simulink model "ES004A_PwrUpSeq"  (R2013b)
settings: Solver=FixedStepDiscrete  SolverMode=SingleTasking  StartTime=0.0  StopTime=1  FixedStep=0.002  RelTol=1e-3
undefined symbols (not defined in the file): ELECGLBPRM_STRTUPSTCURRMEASWRMININTESTSTRT_CNT_U08, ELECGLBPRM_STRTUPSTDI_CNT_U08, ELECGLBPRM_STRTUPSTFLSMEMININSTRT_CNT_U08, ELECGLBPRM_STRTUPSTMTRDRVRININSTRT_CNT_U08, ELECGLBPRM_STRTUPSTPWRDISCNCTATESTSTRT_CNT_U08, ELECGLBPRM_STRTUPSTPWRDISCNCTBTESTSTRT_CNT_U08, ELECGLBPRM_STRTUPSTTMPLMONININTESTSTRT_CNT_U08, ELECGLBPRM_STRTUPSTWARMININCMPL_CNT_U08, PWRTURNOFFCTRLTHD_CNT_U08, sigbuilder_block
libraries: simulink x3
(part 1 of 2)
settings Model: Creator=BZ9NJH  LastModifiedBy=TZBSJD
settings SolverCC: AutoInsertRateTranBlk=on  InsertRTBMode=Always
settings DataIOCC: LimitDataPoints=off  SaveFormat=Structure  ReturnWorkspaceOutputs=on
settings OptimizationCC: BlockReduction=off  InlineParams=on  ZeroExternalMemoryAtStartup=off  ZeroInternalMemoryAtStartup=off  OptimizeModelRefInitCode=on  LifeSpan=1
settings DebuggingCC: SignalInfNanChecking=error  SignalRangeChecking=warning  UnderspecifiedInitializationDetection=Simplified  SolverPrmCheckMsg=error  InheritedTsInSrcMsg=error  DiscreteInheritContinuousMsg=error  SingleTaskRateTransMsg=error  TasksWithSamePriorityMsg=error  SigSpecEnsureSampleTimeMsg=error  CheckMatrixSingularityMsg=error  IntegerOverflowMsg=none  ParameterUnderflowMsg=error  ParameterPrecisionLossMsg=error  ParameterTunabilityLossMsg=error  FixptConstUnderflowMsg=warning  FixptConstOverflowMsg=warning  VectorMatrixConversionMsg=error  SignalLabelMismatchMsg=error  UnconnectedInputMsg=error  UnconnectedOutputMsg=error  UnconnectedLineMsg=error  SFcnCompatibilityMsg=error  UniqueDataStoreMsg=warning  BusObjectLabelMismatch=error  RootOutportRequireBusObject=error  AssertControl=DisableAll  ModelReferenceIOMsg=error  ModelReferenceVersionMismatchMessage=warning  ModelReferenceIOMismatchMessage=error  ModelReferenceCSMismatchMessage=warning  ModelReferenceDataLoggingMessage=error  StateNameClashWarn=warning  StrictBusMsg=ErrorOnBusTreatedAsVector  NonBusSignalsTreatedAsBus=error  SFUnexpectedBacktrackingDiag=error  SFInvalidInputDataAccessInChartInitDiag=error  SFNoUnconditionalDefaultTransitionDiag=error  SFTransitionOutsideNaturalParentDiag=error  SFUnconditionalTransitionShadowingDiag=error  SFUndirectedBroadcastEventsDiag=error
settings ModelReferenceCC: ModelReferenceNumInstancesAllowed=Single
settings RTWCC: SystemTargetFile=autosar.tlc  GenCodeOnly=on  TemplateMakefile=ert_default_tmf  Description=AUTOSAR  GenerateReport=on  ProcessScript=autosar_make_rtw_hook  LaunchReport=on
settings CodeAppCC: GenerateComments=off  IgnoreCustomStorageClasses=off  CustomSymbolStrType=$N$R$M  CustomSymbolStrBlkIO=$N$M  SimulinkBlockComments=off
settings STFCustomTargetCC: ParMdlRefBuildCompliant=on  CompOptLevelCompliant=on  IncludeMdlTerminateFcn=off  CombineOutputUpdateFcns=on  SuppressErrorStatus=on  ERTFirstTimeCompliant=on  ERTCustomFileBanners=on  SupportNonFinite=off  SupportComplex=off  SupportContinuousTime=off  SupportNonInlinedSFcns=off  MATLABClassNameForMDSCustomization=Simulink.SoftwareTarget.ERTCustomization  AutosarCompliant=on  GRTInterface=off  SystemTargetFile=autosar.tlc
settings ERTTargetCC: CodeReplacementLibrary=ANSI_C  ConcurrentExecutionCompliant=off  IncludeMdlTerminateFcn=off  SuppressErrorStatus=on  SupportNonFinite=off  SupportComplex=off  ModelStepFunctionPrototypeControlCompliant=off  CPPClassGenCompliant=off  AutosarCompliant=on  InlinedParameterPlacement=NonHierarchical  ERTCustomFileTemplate=example_file_process.tlc  EnableUserReplacementTypes=on

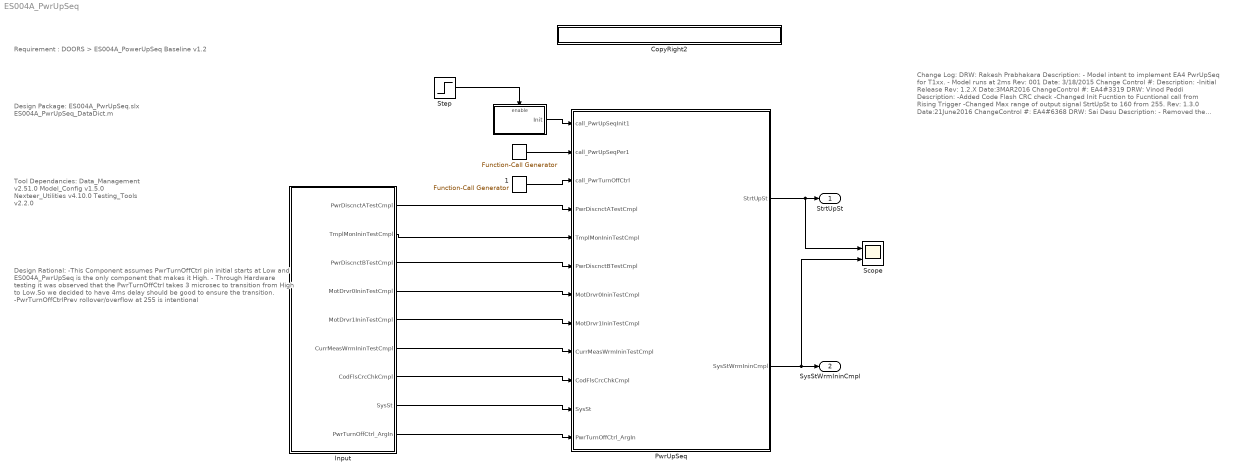
== system ES004A_PwrUpSeq ==
  note: Tool Dependancies:
      |
      | Data_Management v2.51.0
      | Model_Config v1.5.0
      | Nexteer_Utilities v4.10.0
      | Testing_Tools v2.2.0
  note: Design Package:
      |
      | ES004A_PwrUpSeq.slx
      | ES004A_PwrUpSeq_DataDict.m
  note: Requirement :
      |
      | DOORS > ES004A_PowerUpSeq Baseline v1.2
  note: Change Log:
      |
      | DRW: Rakesh Prabhakara
      | Description:
      | - Model intent to implement EA4 PwrUpSeq for T1xx.
      | - Model runs at 2ms
      |
      |
      | Rev: 001
      | Date: 3/18/2015
      | Change Control #:
      |
      | Description:
      | -Initial Release
      |
      | Rev: 1.2.X
      | Date:3MAR2016
      | ChangeControl #: EA4#3319
      | DRW: Vinod Peddi
      | Description:
      | -Added Code Flash CRC check
      | -Changed Init Fucntion to Fucntional call from Rising Trigger
      | -Changed Max range of output signal StrtUpSt to 160 from 255.
      |
      | Rev: 1.3.0
      | Date:21June2016
      | ChangeControl #: EA4#6368
      | DRW: Sai Desu
      | Description:
      | - Removed the StateFlow.
      |
      | Rev: 1.4.0
      | Date:7/12/2016
      | ChangeControl #: 	EA4#6487
      | DRW: Vinod Peddi
      | Description:
      | - Added MotDrv0IninTestCmpl and MotDrv1IninTestCmpl
      | -(Accounting for the changes in the Gate Drive FDDs)
      |
      | Rev: 1.5.0
      | Date:12/02/2016
      | ChangeControl #: 	EA4#8720
      | DRW: Sai Desu
      | Description:
      | - Added  logic in per1 to get TODpin to High state
      | - Added a new constant TURNOFFDLYTHD_CNT_U08 and new PIM PwrTurnOffCtrlPrev
      | -Added a new server for  PwrTurnOffCtrl pin control.
  note: Design Rational:
      | -This Component assumes PwrTurnOffCtrl pin
      | initial starts at Low and ES004A_PwrUpSeq
      | is the only component that makes it High.
      | - Through Hardware testing it was observed that
      | the PwrTurnOffCtrl takes 3 microsec to transition
      | from High to Low.So we decided to have 4ms delay
      | should be good to ensure the transition.
      | -PwrTurnOffCtrlPrev rollover/overflow at 255 is intentional
  "   " : simulink/Ports & Subsystems/Function-Call Generator  sample_time=0.002  numberOfIterations=1
  "    " : Subsystem  TreatAsAtomicUnit=on
  "   1" : simulink/Ports & Subsystems/Function-Call Generator  sample_time=0.002  numberOfIterations=1
  CopyRight2 : Subsystem  Description=|  mask(Copyright Information){none=on}
      | Copyright info block.                                               
      |                                                                     
      | Place copyright information at the top of every subsystem in design.
      mask prompts: none "No parameters"
      mask help: Place copyright information at the top of every subsystem in design.
      mask Display:
      | NxtrConf = 'Nexteer Confidential';
      | 
      | sys = bdroot; %handle for the current model ("system")
      | first = get_param(sys,'Created');
      | first = first(end-3:end);  %year is last four digits
      | 
      | last = get_param(sys,'LastModifiedDate');
      | if isempty(last)
      |     last = datestr(now,'yyyy');
      | else
      |     last = last(end-3:end);
      | end
      | 
      | if strcmp(first,last)
      |     fprintf('%s -- Copyright %s Nexteer',NxtrConf,first)
      | else
      |     fprintf('%s -- %s%s- %s Nexteer',NxtrConf,char(169),first,last)
      | end
  Input : Subsystem
      settings: AttributesFormatString=FOR SIMULATION ONLY
  PwrUpSeq : Subsystem  RequirementInfo={} %GIDa_35cfe924_8c92_4195_bef3_596e1ba51ef0
  Scope : Scope  NumInputPorts=2
      settings: YMin=-5~-5  YMax=5~5
  Step : Step  Before=1  After=0  SampleTime=0
  StrtUpSt : Outport
  SysStWrmIninCmpl : Outport  Port=2
  wires:
  "   "/1 -> PwrUpSeq/2(call_PwrUpSeqPer1)
  "    "/1(Init) -> PwrUpSeq/1(call_PwrUpSeqInit1)
  PwrUpSeq/1(StrtUpSt) -> StrtUpSt/1, Scope/1
  PwrUpSeq/2(SysStWrmIninCmpl) -> Scope/2, SysStWrmIninCmpl/1
  Step/1 -> "    "/Enable
  Input/1(PwrDiscnctATestCmpl) -> PwrUpSeq/4(PwrDiscnctATestCmpl)
  Input/2("TmplMonIninTestCmpl ") -> PwrUpSeq/5(TmplMonIninTestCmpl)
  Input/3(PwrDiscnctBTestCmpl) -> PwrUpSeq/6(PwrDiscnctBTestCmpl)
  Input/4(MotDrvr0IninTestCmpl) -> PwrUpSeq/7(MotDrvr0IninTestCmpl)
  Input/6(CurrMeasWrmIninTestCmpl) -> PwrUpSeq/9(CurrMeasWrmIninTestCmpl)
  Input/7(CodFlsCrcChkCmpl) -> PwrUpSeq/10(CodFlsCrcChkCmpl)
  Input/8(SysSt) -> PwrUpSeq/11(SysSt)
  Input/5(MotDrvr1IninTestCmpl) -> PwrUpSeq/8(MotDrvr1IninTestCmpl)
  "   1"/1 -> PwrUpSeq/3(call_PwrTurnOffCtrl)
  Input/9(PwrTurnOffCtrl_ArgIn) -> PwrUpSeq/12(PwrTurnOffCtrl_ArgIn)

== system ES004A_PwrUpSeq/     ==
  Enable : EnablePort
  CopyRight2 : Subsystem  Description=|  mask(Copyright Information){none=on}
      | Copyright info block.                                               
      |                                                                     
      | Place copyright information at the top of every subsystem in design.
      mask prompts: none "No parameters"
      mask help: Place copyright information at the top of every subsystem in design.
      mask Display:
      | NxtrConf = 'Nexteer Confidential';
      | 
      | sys = bdroot; %handle for the current model ("system")
      | first = get_param(sys,'Created');
      | first = first(end-3:end);  %year is last four digits
      | 
      | last = get_param(sys,'LastModifiedDate');
      | if isempty(last)
      |     last = datestr(now,'yyyy');
      | else
      |     last = last(end-3:end);
      | end
      | 
      | if strcmp(first,last)
      |     fprintf('%s -- Copyright %s Nexteer',NxtrConf,first)
      | else
      |     fprintf('%s -- %s%s- %s Nexteer',NxtrConf,char(169),first,last)
      | end
  call_GateDrvCtrlInit1 : simulink/Ports & Subsystems/Function-Call Generator  sample_time=0  numberOfIterations=1
  Init : Outport
  wires:
  call_GateDrvCtrlInit1/1 -> Init/1

== system ES004A_PwrUpSeq/CopyRight2 ==

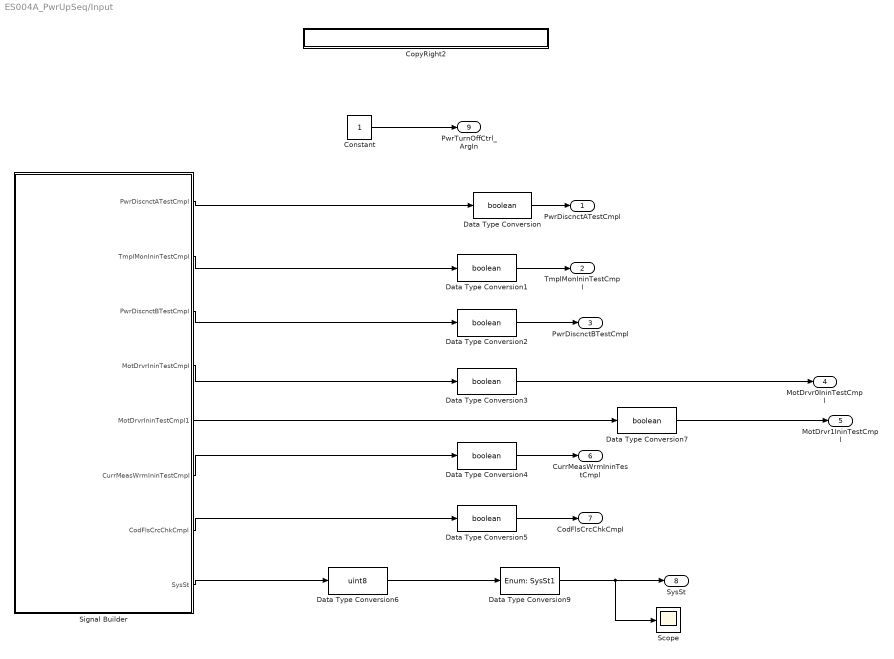
== system ES004A_PwrUpSeq/Input ==
  Constant : Constant  OutDataTypeStr=boolean
  CopyRight2 : Subsystem  Description=|  mask(Copyright Information){none=on}
      | Copyright info block.                                               
      |                                                                     
      | Place copyright information at the top of every subsystem in design.
      mask prompts: none "No parameters"
      mask help: Place copyright information at the top of every subsystem in design.
      mask Display:
      | NxtrConf = 'Nexteer Confidential';
      | 
      | sys = bdroot; %handle for the current model ("system")
      | first = get_param(sys,'Created');
      | first = first(end-3:end);  %year is last four digits
      | 
      | last = get_param(sys,'LastModifiedDate');
      | if isempty(last)
      |     last = datestr(now,'yyyy');
      | else
      |     last = last(end-3:end);
      | end
      | 
      | if strcmp(first,last)
      |     fprintf('%s -- Copyright %s Nexteer',NxtrConf,first)
      | else
      |     fprintf('%s -- %s%s- %s Nexteer',NxtrConf,char(169),first,last)
      | end
  Data Type Conversion{,1..5,7} (7 alike) : DataTypeConversion  OutDataTypeStr=boolean
  Data Type Conversion6 : DataTypeConversion  OutDataTypeStr=uint8
  Data Type Conversion9 : DataTypeConversion  OutDataTypeStr=Enum: SysSt1
      settings: AttributesFormatString=%<BlockType>
  Scope : Scope
  Signal Builder : Subsystem  Tag=STV Subsys  LoadFcn=sigbuilder_block('load');  StartFcn=sigbuilder_block('start');  StopFcn=sigbuilder_block('stop');  ClipboardFcn=sigbuilder_block('clipboard');  mask(Sigbuilder block){}
      mask help: Simulink:masks:SigbuilderBlock_MD
      mask init:
      | if ~strcmp(get_param(bdroot(gcbh),'SimulationStatus'),'stopped') tuvar = sigbuilder_block('maskInit'); end
      settings: CopyFcn=sigbuilder_block('copy');  DeleteFcn=sigbuilder_block('delete');  ModelCloseFcn=sigbuilder_block('modelClose');  PreSaveFcn=sigbuilder_block('preSave');  PauseFcn=sigbuilder_block('pause');  ContinueFcn=sigbuilder_block('continue');  NameChangeFcn=sigbuilder_block('namechange');  OpenFcn=sigbuilder_block('open',[-1024.5 11.25 1024.5 519 ]);  CloseFcn=sigbuilder_block('close');
      mask Display: plot(0, 0, 100, 100,[2, 2, 32, 32, 2], [68, 8, 8, 68, 68],[32, 2], [38, 38], [32, 19, 2],[53, 60, 44], [32, 17, 17, 2],[16, 16, 31, 31]);txt = getActiveGroup(gcbh);text(2, 100, txt,'verticalAlignment', 'top');
  PwrDiscnctATestCmpl : Outport
  "TmplMonIninTestCmpl " : Outport  Port=2
  PwrDiscnctBTestCmpl : Outport  Port=3
  MotDrvr0IninTestCmpl : Outport  Port=4
  MotDrvr1IninTestCmpl : Outport  Port=5
  CurrMeasWrmIninTestCmpl : Outport  Port=6
  CodFlsCrcChkCmpl : Outport  Port=7
  SysSt : Outport  Port=8
  PwrTurnOffCtrl_ArgIn : Outport  Port=9
  wires:
  Data Type Conversion/1 -> PwrDiscnctATestCmpl/1
  Data Type Conversion1/1 -> "TmplMonIninTestCmpl "/1
  Data Type Conversion2/1 -> PwrDiscnctBTestCmpl/1
  Data Type Conversion3/1 -> MotDrvr0IninTestCmpl/1
  Data Type Conversion4/1 -> CurrMeasWrmIninTestCmpl/1
  Data Type Conversion5/1 -> CodFlsCrcChkCmpl/1
  Data Type Conversion6/1 -> Data Type Conversion9/1
  Data Type Conversion9/1 -> Scope/1, SysSt/1
  Signal Builder/1(PwrDiscnctATestCmpl) -> Data Type Conversion/1
  Signal Builder/2(TmplMonIninTestCmpl) -> Data Type Conversion1/1
  Signal Builder/3(PwrDiscnctBTestCmpl) -> Data Type Conversion2/1
  Signal Builder/4(MotDrvrIninTestCmpl) -> Data Type Conversion3/1
  Signal Builder/6(CurrMeasWrmIninTestCmpl) -> Data Type Conversion4/1
  Signal Builder/7(CodFlsCrcChkCmpl) -> Data Type Conversion5/1
  Signal Builder/8(SysSt) -> Data Type Conversion6/1
  Signal Builder/5(MotDrvrIninTestCmpl1) -> Data Type Conversion7/1
  Data Type Conversion7/1 -> MotDrvr1IninTestCmpl/1
  Constant/1 -> PwrTurnOffCtrl_ArgIn/1

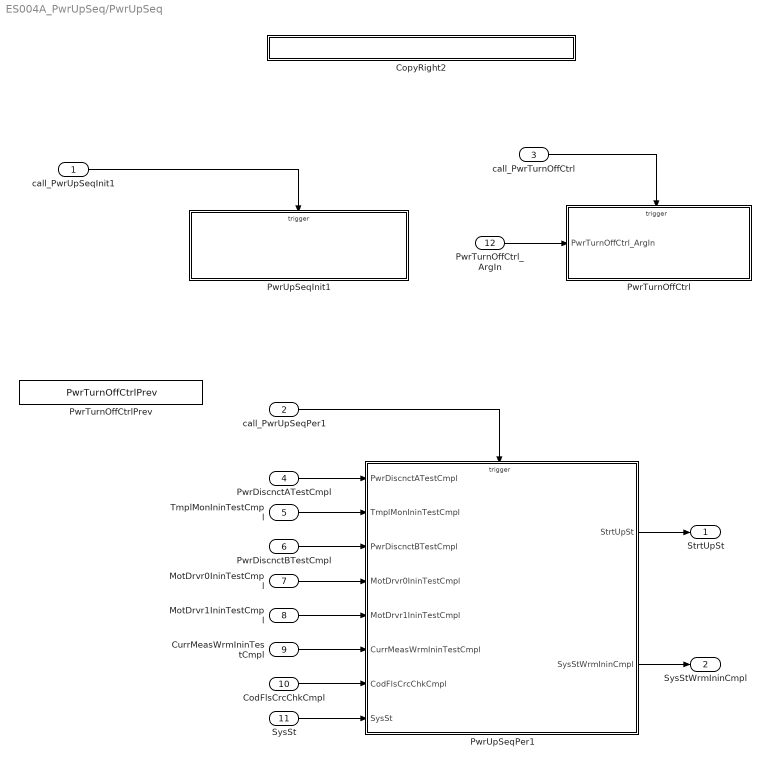
== system ES004A_PwrUpSeq/PwrUpSeq ==
  call_PwrUpSeqInit1 : Inport
  call_PwrUpSeqPer1 : Inport  Port=2
  call_PwrTurnOffCtrl : Inport  Port=3
  PwrDiscnctATestCmpl : Inport  RequirementInfo={} %GIDa_446bf28d_326e_4d71_9178_cb8879d17d30  Port=4
  TmplMonIninTestCmpl : Inport  RequirementInfo={} %GIDa_051ede06_809d_4a6b_ab11_6adf88300e4f  Port=5
  PwrDiscnctBTestCmpl : Inport  RequirementInfo={} %GIDa_4ad84e80_8ac9_4153_860d_30c67dab3eca  Port=6
  MotDrvr0IninTestCmpl : Inport  RequirementInfo={} %GIDa_14d41728_be18_48b9_a298_4b5d0108ece5  Port=7
  MotDrvr1IninTestCmpl : Inport  RequirementInfo="{}  %GIDa_c04dc9a0_694b_4c78_818e_03ab0f3abce0"  Port=8
  CurrMeasWrmIninTestCmpl : Inport  RequirementInfo={} %GIDa_d2f15d57_cae9_46da_aa94_3e87a93d3250  Port=9
  CodFlsCrcChkCmpl : Inport  RequirementInfo={} %GIDa_a8ee0d48_f2b0_430a_b961_b39c593c106a  Port=10
  SysSt : Inport  RequirementInfo={} %GIDa_cd61f2f6_0fac_48ad_93c3_ac49d9e424fd  Port=11
  PwrTurnOffCtrl_ArgIn : Inport  Port=12
  CopyRight2 : Subsystem  Description=|  mask(Copyright Information){none=on}
      | Copyright info block.                                               
      |                                                                     
      | Place copyright information at the top of every subsystem in design.
      mask prompts: none "No parameters"
      mask help: Place copyright information at the top of every subsystem in design.
      mask Display:
      | NxtrConf = 'Nexteer Confidential';
      | 
      | sys = bdroot; %handle for the current model ("system")
      | first = get_param(sys,'Created');
      | first = first(end-3:end);  %year is last four digits
      | 
      | last = get_param(sys,'LastModifiedDate');
      | if isempty(last)
      |     last = datestr(now,'yyyy');
      | else
      |     last = last(end-3:end);
      | end
      | 
      | if strcmp(first,last)
      |     fprintf('%s -- Copyright %s Nexteer',NxtrConf,first)
      | else
      |     fprintf('%s -- %s%s- %s Nexteer',NxtrConf,char(169),first,last)
      | end
  PwrTurnOffCtrl : Subsystem  RequirementInfo={} %GIDa_2ddf7215_35b5_4bad_85c7_079bbc552366
  PwrTurnOffCtrlPrev : DataStoreMemory  DataStoreName=PwrTurnOffCtrlPrev  StateMustResolveToSignalObject=on
  PwrUpSeqInit1 : Subsystem
  PwrUpSeqPer1 : Subsystem  TreatAsAtomicUnit=on
  StrtUpSt : Outport  RequirementInfo={} %GIDa_a09a46f2_e758_4418_b300_e7ddefb852d6
  SysStWrmIninCmpl : Outport  RequirementInfo={} %GIDa_a94a2f61_8623_40ca_87d4_e2cd322971b0  Port=2
  wires:
  call_PwrUpSeqPer1/1 -> PwrUpSeqPer1/Trigger
  TmplMonIninTestCmpl/1 -> PwrUpSeqPer1/2(TmplMonIninTestCmpl)
  PwrDiscnctATestCmpl/1 -> PwrUpSeqPer1/1(PwrDiscnctATestCmpl)
  PwrDiscnctBTestCmpl/1 -> PwrUpSeqPer1/3(PwrDiscnctBTestCmpl)
  MotDrvr0IninTestCmpl/1 -> PwrUpSeqPer1/4(MotDrvr0IninTestCmpl)
  PwrUpSeqPer1/2(SysStWrmIninCmpl) -> SysStWrmIninCmpl/1
  PwrUpSeqPer1/1(StrtUpSt) -> StrtUpSt/1
  CurrMeasWrmIninTestCmpl/1 -> PwrUpSeqPer1/6("CurrMeasWrmIninTestCmpl ")
  SysSt/1 -> PwrUpSeqPer1/8(SysSt)
  CodFlsCrcChkCmpl/1 -> PwrUpSeqPer1/7(CodFlsCrcChkCmpl)
  call_PwrUpSeqInit1/1 -> PwrUpSeqInit1/Trigger
  MotDrvr1IninTestCmpl/1 -> PwrUpSeqPer1/5(MotDrvr1IninTestCmpl)
  call_PwrTurnOffCtrl/1 -> PwrTurnOffCtrl/Trigger
  PwrTurnOffCtrl_ArgIn/1 -> PwrTurnOffCtrl/1(PwrTurnOffCtrl_ArgIn)

== system ES004A_PwrUpSeq/    /CopyRight2 ==

== system ES004A_PwrUpSeq/Input/CopyRight2 ==

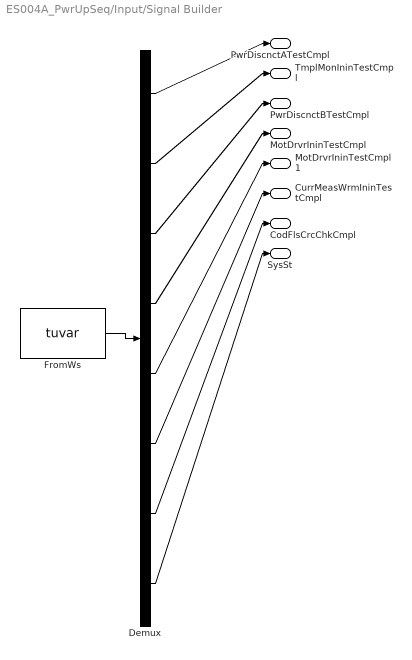
== system ES004A_PwrUpSeq/Input/Signal Builder ==
  Demux : Demux  Tag=STV Demux  Outputs=8
  FromWs : FromWorkspace  Tag=STV FromWs  VariableName=tuvar  SampleTime=0
      SigBuilderData=|
      | common.afterFinalStr = 'Extrapolate'
      | common.sampleTime = 0
      | dataSet(1).timeRange = [0 1]
      | dataSet(1).name = 'Ano Result'
      | dataSet(2).timeRange = [0 1]
      | dataSet(2).name = 'Loop Check'
      | dataSet(3).timeRange = [0 1]
      | dataSet(3).name = 'Loop Check1'
      | dataSet(4).timeRange = [0 1]
      | dataSet(4).name = 'Loop Check2'
      | sbobj.Groups(1).Name = 'Ano Result'
      | sbobj.Groups(1).Signals(1).Name = 'PwrDiscnctATestCmpl'
      | sbobj.Groups(1).Signals(1).XData = [0 0.19 0.62 1]
      | sbobj.Groups(1).Signals(1).YData = [1 1 1 1]
      | sbobj.Groups(1).Signals(2).Name = 'TmplMonIninTestCmpl'
      | sbobj.Groups(1).Signals(2).XData = [0 0.36 0.88 1]
      | sbobj.Groups(1).Signals(2).YData = [1 1 1 1]
      | sbobj.Groups(1).Signals(3).Name = 'PwrDiscnctBTestCmpl'
      | sbobj.Groups(1).Signals(3).XData = [0 0.53 1]
      | sbobj.Groups(1).Signals(3).YData = [1 1 1]
      | sbobj.Groups(1).Signals(4).Name = 'MotDrvrIninTestCmpl'
      | sbobj.Groups(1).Signals(4).XData = [0 0.7 1]
      | sbobj.Groups(1).Signals(4).YData = [1 1 1]
      | sbobj.Groups(1).Signals(5).Name = 'MotDrvrIninTestCmpl1'
      | sbobj.Groups(1).Signals(5).XData = [0 0.4 0.4 0.6 0.6 1]
      | sbobj.Groups(1).Signals(5).YData = [0 0 1 1 0 0]
      | sbobj.Groups(1).Signals(6).Name = 'CurrMeasWrmIninTestCmpl'
      | sbobj.Groups(1).Signals(6).XData = [0 0.92 1]
      | sbobj.Groups(1).Signals(6).YData = [1 1 1]
      | sbobj.Groups(1).Signals(7).Name = 'CodFlsCrcChkCmpl'
      | sbobj.Groups(1).Signals(7).XData = [0 1]
      | sbobj.Groups(1).Signals(7).YData = [1 1]
      | sbobj.Groups(1).Signals(8).Name = 'SysSt'
      | sbobj.Groups(1).Signals(8).XData = [0 1]
      | sbobj.Groups(1).Signals(8).YData = [3 3]
      | sbobj.Groups(1).TimeRange = [0 1]
      | sbobj.Groups(2).Name = 'Loop Check'
      | sbobj.Groups(2).Signals(1).Name = 'PwrDiscnctATestCmpl'
      | sbobj.Groups(2).Signals(1).XData = [0 0.078 0.078 0.156 0.156 0.19 0.62 1]
      | sbobj.Groups(2).Signals(1).YData = [1 1 0 0 1 1 1 1]
      | sbobj.Groups(2).Signals(2).Name = 'TmplMonIninTestCmpl'
      | sbobj.Groups(2).Signals(2).XData = [0 0.3 0.3 0.88 1]
      | sbobj.Groups(2).Signals(2).YData = [0 0 1 1 1]
      | sbobj.Groups(2).Signals(3).Name = 'PwrDiscnctBTestCmpl'
      | sbobj.Groups(2).Signals(3).XData = [0 0.4 0.4 1]
      | sbobj.Groups(2).Signals(3).YData = [0 0 1 1]
      | sbobj.Groups(2).Signals(4).Name = 'MotDrvrIninTestCmpl'
      | sbobj.Groups(2).Signals(4).XData = [0 0.501 0.501 1]
      | sbobj.Groups(2).Signals(4).YData = [0 0 1 1]
      | sbobj.Groups(2).Signals(5).Name = 'MotDrvrIninTestCmpl1'
      | sbobj.Groups(2).Signals(5).XData = [0 0.6 0.6 1]
      | sbobj.Groups(2).Signals(5).YData = [0 0 1 1]
      | sbobj.Groups(2).Signals(6).Name = 'CurrMeasWrmIninTestCmpl'
      | sbobj.Groups(2).Signals(6).XData = [0 0.7 0.7 1]
      | sbobj.Groups(2).Signals(6).YData = [0 0 1 1]
      | sbobj.Groups(2).Signals(7).Name = 'CodFlsCrcChkCmpl'
      | sbobj.Groups(2).Signals(7).XData = [0 0.8 0.8 1]
      | sbobj.Groups(2).Signals(7).YData = [0 0 1 1]
      | sbobj.Groups(2).Signals(8).Name = 'SysSt'
      | sbobj.Groups(2).Signals(8).XData = [0 0.045 0.045 0.098 0.098 0.331 0.331 0.359 0.359 0.522 0.522 0.562 0.562 1]
      | sbobj.Groups(2).Signals(8).YData = [0 0 1 1 3 3 1 1 3 3 2 2 3 3]
      | sbobj.Groups(2).TimeRange = [0 1]
      | sbobj.Groups(3).Name = 'Loop Check1'
      | sbobj.Groups(3).Signals(1).Name = 'PwrDiscnctATestCmpl'
      | sbobj.Groups(3).Signals(1).XData = [0 0.078 0.156 0.156 0.19 0.62 1]
      | sbobj.Groups(3).Signals(1).YData = [0 0 0 1 1 1 1]
      | sbobj.Groups(3).Signals(2).Name = 'TmplMonIninTestCmpl'
      | sbobj.Groups(3).Signals(2).XData = [0 0.2 0.2 0.88 1]
      | sbobj.Groups(3).Signals(2).YData = [0 0 1 1 1]
      | sbobj.Groups(3).Signals(3).Name = 'PwrDiscnctBTestCmpl'
      | sbobj.Groups(3).Signals(3).XData = [0 0.234 0.234 1]
      | sbobj.Groups(3).Signals(3).YData = [0 0 1 1]
      | sbobj.Groups(3).Signals(4).Name = 'MotDrvrIninTestCmpl'
      | sbobj.Groups(3).Signals(4).XData = [0 0.272 0.272 1]
      | sbobj.Groups(3).Signals(4).YData = [0 0 1 1]
      | sbobj.Groups(3).Signals(5).Name = 'MotDrvrIninTestCmpl1'
      | sbobj.Groups(3).Signals(5).XData = [0 0.274 1]
      | sbobj.Groups(3).Signals(5).YData = [0 0 0]
      | sbobj.Groups(3).Signals(6).Name = 'CurrMeasWrmIninTestCmpl'
      | sbobj.Groups(3).Signals(6).XData = [0 0.308 0.308 1]
      | sbobj.Groups(3).Signals(6).YData = [0 0 1 1]
      | sbobj.Groups(3).Signals(7).Name = 'CodFlsCrcChkCmpl'
      | sbobj.Groups(3).Signals(7).XData = [0 0.34 0.34 1]
      | sbobj.Groups(3).Signals(7).YData = [0 0 1 1]
      | sbobj.Groups(3).Signals(8).Name = 'SysSt'
      | sbobj.Groups(3).Signals(8).XData = [0 0.045 0.098 0.331 0.359 0.444 1]
      | sbobj.Groups(3).Signals(8).YData = [3 3 3 3 3 3 3]
      | sbobj.Groups(3).TimeRange = [0 1]
      | sbobj.Groups(4).Name = 'Loop Check2'
      | sbobj.Groups(4).Signals(1).Name = 'PwrDiscnctATestCmpl'
      | sbobj.Groups(4).Signals(1).XData = [0 0.078 0.156 0.156 0.19 0.62 1]
      | sbobj.Groups(4).Signals(1).YData = [0 0 0 1 1 1 1]
      | sbobj.Groups(4).Signals(2).Name = 'TmplMonIninTestCmpl'
      | sbobj.Groups(4).Signals(2).XData = [0 0.2 0.2 0.88 1]
      | sbobj.Groups(4).Signals(2).YData = [0 0 1 1 1]
      | sbobj.Groups(4).Signals(3).Name = 'PwrDiscnctBTestCmpl'
      | sbobj.Groups(4).Signals(3).XData = [0 0.234 0.234 1]
      | sbobj.Groups(4).Signals(3).YData = [0 0 1 1]
      | sbobj.Groups(4).Signals(4).Name = 'MotDrvrIninTestCmpl'
      | sbobj.Groups(4).Signals(4).XData = [0 0.272 0.272 1]
      | sbobj.Groups(4).Signals(4).YData = [0 0 1 1]
      | sbobj.Groups(4).Signals(5).Name = 'MotDrvrIninTestCmpl1'
      | sbobj.Groups(4).Signals(5).XData = [0 0.333 0.333 1]
      | sbobj.Groups(4).Signals(5).YData = [0 0 1 1]
      | sbobj.Groups(4).Signals(6).Name = 'CurrMeasWrmIninTestCmpl'
      | sbobj.Groups(4).Signals(6).XData = [0 0.308 0.308 1]
      | sbobj.Groups(4).Signals(6).YData = [0 0 1 1]
      | sbobj.Groups(4).Signals(7).Name = 'CodFlsCrcChkCmpl'
      | sbobj.Groups(4).Signals(7).XData = [0 0.34 0.34 1]
      | sbobj.Groups(4).Signals(7).YData = [0 0 1 1]
      | sbobj.Groups(4).Signals(8).Name = 'SysSt'
      | sbobj.Groups(4).Signals(8).XData = [0 0.045 0.098 0.331 0.359 0.359 0.444 0.444 1]
      | sbobj.Groups(4).Signals(8).YData = [3 3 3 3 3 0 0 2 2]
      | sbobj.Groups(4).TimeRange = [0 1]
  PwrDiscnctATestCmpl : Outport  Tag=STV Outport
  TmplMonIninTestCmpl : Outport  Tag=STV Outport  Port=2
  PwrDiscnctBTestCmpl : Outport  Tag=STV Outport  Port=3
  MotDrvrIninTestCmpl : Outport  Tag=STV Outport  Port=4
  MotDrvrIninTestCmpl1 : Outport  Tag=STV Outport  Port=5
  CurrMeasWrmIninTestCmpl : Outport  Tag=STV Outport  Port=6
  CodFlsCrcChkCmpl : Outport  Tag=STV Outport  Port=7
  SysSt : Outport  Tag=STV Outport  Port=8
  wires:
  FromWs/1 -> Demux/1
  Demux/1 -> PwrDiscnctATestCmpl/1
  Demux/2 -> TmplMonIninTestCmpl/1
  Demux/3 -> PwrDiscnctBTestCmpl/1
  Demux/4 -> MotDrvrIninTestCmpl/1
  Demux/5 -> MotDrvrIninTestCmpl1/1
  Demux/6 -> CurrMeasWrmIninTestCmpl/1
  Demux/7 -> CodFlsCrcChkCmpl/1
  Demux/8 -> SysSt/1

== system ES004A_PwrUpSeq/PwrUpSeq/CopyRight2 ==

== system ES004A_PwrUpSeq/PwrUpSeq/PwrTurnOffCtrl ==
  note: Note:
      | It is a function call for PIN P0_13
  PwrTurnOffCtrl_ArgIn : Inport
  function : TriggerPort  TriggerType=function-call
  CopyRight2 : Subsystem  Description=|  mask(Copyright Information){none=on}
      | Copyright info block.                                               
      |                                                                     
      | Place copyright information at the top of every subsystem in design.
      mask prompts: none "No parameters"
      mask help: Place copyright information at the top of every subsystem in design.
      mask Display:
      | NxtrConf = 'Nexteer Confidential';
      | 
      | sys = bdroot; %handle for the current model ("system")
      | first = get_param(sys,'Created');
      | first = first(end-3:end);  %year is last four digits
      | 
      | last = get_param(sys,'LastModifiedDate');
      | if isempty(last)
      |     last = datestr(now,'yyyy');
      | else
      |     last = last(end-3:end);
      | end
      | 
      | if strcmp(first,last)
      |     fprintf('%s -- Copyright %s Nexteer',NxtrConf,first)
      | else
      |     fprintf('%s -- %s%s- %s Nexteer',NxtrConf,char(169),first,last)
      | end
  IoHwAb_SetGpioPwrTurnOffCtrl : Subsystem  RequirementInfo={} %GIDa_63a85690_40db_495f_9f73_413351781123  TreatAsAtomicUnit=on
  wires:
  PwrTurnOffCtrl_ArgIn/1 -> IoHwAb_SetGpioPwrTurnOffCtrl/1(PinSt)

== system ES004A_PwrUpSeq/PwrUpSeq/PwrUpSeqInit1 ==
  note: Do Nothing
  function : TriggerPort  TriggerType=function-call
  CopyRight2 : Subsystem  Description=|  mask(Copyright Information){none=on}
      | Copyright info block.                                               
      |                                                                     
      | Place copyright information at the top of every subsystem in design.
      mask prompts: none "No parameters"
      mask help: Place copyright information at the top of every subsystem in design.
      mask Display:
      | NxtrConf = 'Nexteer Confidential';
      | 
      | sys = bdroot; %handle for the current model ("system")
      | first = get_param(sys,'Created');
      | first = first(end-3:end);  %year is last four digits
      | 
      | last = get_param(sys,'LastModifiedDate');
      | if isempty(last)
      |     last = datestr(now,'yyyy');
      | else
      |     last = last(end-3:end);
      | end
      | 
      | if strcmp(first,last)
      |     fprintf('%s -- Copyright %s Nexteer',NxtrConf,first)
      | else
      |     fprintf('%s -- %s%s- %s Nexteer',NxtrConf,char(169),first,last)
      | end

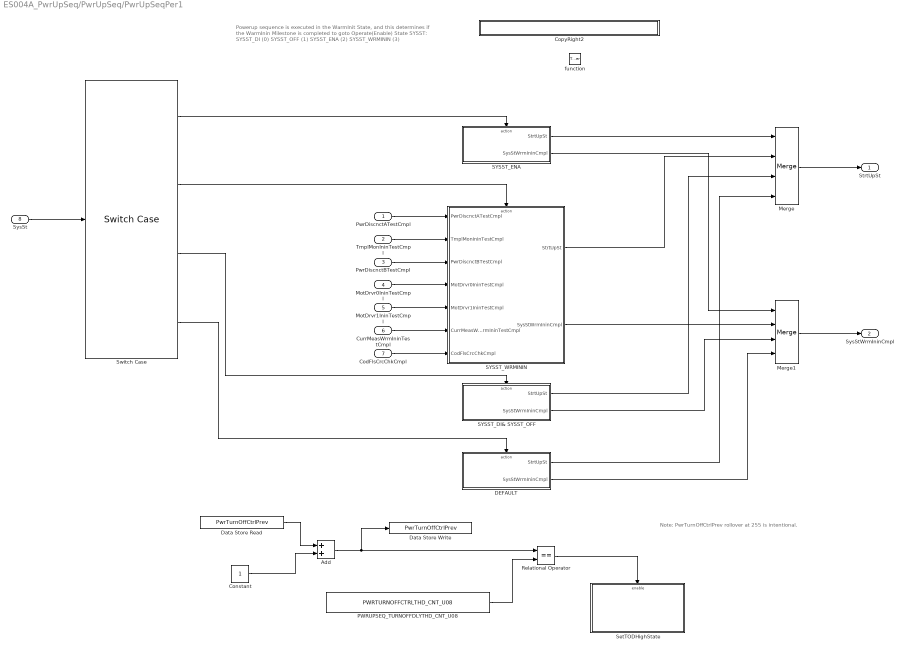
== system ES004A_PwrUpSeq/PwrUpSeq/PwrUpSeqPer1 ==
  note: Note:
      |       PwrTurnOffCtrlPrev rollover at 255 is intentional.
  note: Powerup sequence is executed in the WarmInit State, and this determines
      | if the WarmInin Milestone is completed to goto Operate(Enable) State
      |
      | SYSST:
      |         SYSST_DI               (0)
      |         SYSST_OFF            (1)
      |         SYSST_ENA            (2)
      |         SYSST_WRMININ   (3)
  PwrDiscnctATestCmpl : Inport
  TmplMonIninTestCmpl : Inport  Port=2
  PwrDiscnctBTestCmpl : Inport  Port=3
  MotDrvr0IninTestCmpl : Inport  Port=4
  MotDrvr1IninTestCmpl : Inport  Port=5
  "CurrMeasWrmIninTestCmpl " : Inport  Port=6
  CodFlsCrcChkCmpl : Inport  Port=7
  SysSt : Inport  Port=8
  function : TriggerPort  TriggerType=function-call
  Add : Sum
  Constant : Constant  OutDataTypeStr=uint8
  CopyRight2 : Subsystem  Description=|  mask(Copyright Information){none=on}
      | Copyright info block.                                               
      |                                                                     
      | Place copyright information at the top of every subsystem in design.
      mask prompts: none "No parameters"
      mask help: Place copyright information at the top of every subsystem in design.
      mask Display:
      | NxtrConf = 'Nexteer Confidential';
      | 
      | sys = bdroot; %handle for the current model ("system")
      | first = get_param(sys,'Created');
      | first = first(end-3:end);  %year is last four digits
      | 
      | last = get_param(sys,'LastModifiedDate');
      | if isempty(last)
      |     last = datestr(now,'yyyy');
      | else
      |     last = last(end-3:end);
      | end
      | 
      | if strcmp(first,last)
      |     fprintf('%s -- Copyright %s Nexteer',NxtrConf,first)
      | else
      |     fprintf('%s -- %s%s- %s Nexteer',NxtrConf,char(169),first,last)
      | end
  DEFAULT : Subsystem  TreatAsAtomicUnit=on
  Data Store Read : DataStoreRead  DataStoreName=PwrTurnOffCtrlPrev
  Data Store Write : DataStoreWrite  RequirementInfo={} %GIDa_df37f7ff_d87f_4e77_a2b4_f45c46094d7d  DataStoreName=PwrTurnOffCtrlPrev
  Merge : Merge  Inputs=4
  Merge1 : Merge  Inputs=4
  PWRUPSEQ_TURNOFFDLYTHD_CNT_U08 : Constant  Value=PWRTURNOFFCTRLTHD_CNT_U08
  Relational Operator : RelationalOperator  RequirementInfo={'linktype_rmi_doors' '0000c463 (/ESG Group/FDD Module Requirements/EA4 Specific/ES004A_PowerUpSeq)' '#ES004A_113' 'true' 'REQ: ES004A_113' '' } %GIDa_b6b0ea83_391c_4afc_bd1a_4830717992c4  Operator===  OutDataTypeStr=boolean
  SYSST_DI& SYSST_OFF : Subsystem  RequirementInfo="{'linktype_rmi_doors' '0000c463 (/ESG Group/FDD Module Requirements/EA4 Specific/ES004A_PowerUpSeq)' '#ES004A_84' 'true' 'REQ:  ES004A_84' '' } %GIDa_ceeac748_88a8_48cb_815e_66664c5915c7"  TreatAsAtomicUnit=on
  SYSST_ENA : Subsystem  TreatAsAtomicUnit=on
  SYSST_WRMININ : Subsystem  RequirementInfo="{'linktype_rmi_doors' '0000c463 (/ESG Group/FDD Module Requirements/EA4 Specific/ES004A_PowerUpSeq)' '#ES004A_82' 'true' 'REQ:  ES004A_82' '' } %GIDa_50562d96_a11b_4965_9ec2_ad4faf1a6e34"  TreatAsAtomicUnit=on
  "SetTODHighState " : Subsystem  RequirementInfo={'linktype_rmi_doors' '0000c463 (/ESG Group/FDD Module Requirements/EA4 Specific/ES004A_PowerUpSeq)' '#ES004A_113' 'true' 'REQ: ES004A_113' '' } %GIDa_db8fa826_8262_40dd_ba92_80414827086e
  Switch Case : SwitchCase  RequirementInfo="{'linktype_rmi_doors' '0000c463 (/ESG Group/FDD Module Requirements/EA4 Specific/ES004A_PowerUpSeq)' '#ES004A_84' 'true' 'REQ:  ES004A_84' '' } %GIDa_e0e763ba_a867_4216_bd03_69205a1b9b4f"  CaseConditions={SysSt1.SYSST_ENA,SysSt1.SYSST_WRMININ,[SysSt1.SYSST_DI,SysSt1.SYSST_OFF]}
  StrtUpSt : Outport
  SysStWrmIninCmpl : Outport  Port=2
  wires:
  SysSt/1 -> Switch Case/1
  Switch Case/1 -> SYSST_ENA/Action
  Switch Case/2 -> SYSST_WRMININ/Action
  PwrDiscnctATestCmpl/1 -> SYSST_WRMININ/1(PwrDiscnctATestCmpl)
  TmplMonIninTestCmpl/1 -> SYSST_WRMININ/2(TmplMonIninTestCmpl)
  PwrDiscnctBTestCmpl/1 -> SYSST_WRMININ/3(PwrDiscnctBTestCmpl)
  MotDrvr0IninTestCmpl/1 -> SYSST_WRMININ/4(MotDrvr0IninTestCmpl)
  "CurrMeasWrmIninTestCmpl "/1 -> SYSST_WRMININ/6("CurrMeasWrmIninTestCmpl ")
  CodFlsCrcChkCmpl/1 -> SYSST_WRMININ/7(CodFlsCrcChkCmpl)
  Switch Case/4 -> DEFAULT/Action
  Switch Case/3 -> SYSST_DI& SYSST_OFF/Action
  SYSST_WRMININ/1(StrtUpSt) -> Merge/2
  SYSST_ENA/1(StrtUpSt) -> Merge/1
  SYSST_ENA/2(SysStWrmIninCmpl) -> Merge1/1
  SYSST_WRMININ/2(SysStWrmIninCmpl) -> Merge1/2
  Merge/1 -> StrtUpSt/1
  Merge1/1 -> SysStWrmIninCmpl/1
  SYSST_DI& SYSST_OFF/1(StrtUpSt) -> Merge/3
  DEFAULT/1(StrtUpSt) -> Merge/4
  SYSST_DI& SYSST_OFF/2(SysStWrmIninCmpl) -> Merge1/3
  DEFAULT/2(SysStWrmIninCmpl) -> Merge1/4
  MotDrvr1IninTestCmpl/1 -> SYSST_WRMININ/5(MotDrvr1IninTestCmpl)
  Add/1 -> Relational Operator/1, Data Store Write/1
  Constant/1 -> Add/2
  Data Store Read/1 -> Add/1
  PWRUPSEQ_TURNOFFDLYTHD_CNT_U08/1 -> Relational Operator/2
  Relational Operator/1 -> "SetTODHighState "/Enable

== system ES004A_PwrUpSeq/PwrUpSeq/PwrTurnOffCtrl/CopyRight2 ==

== system ES004A_PwrUpSeq/PwrUpSeq/PwrTurnOffCtrl/IoHwAb_SetGpioPwrTurnOffCtrl ==
  PinSt : Inport  OutDataTypeStr=boolean
  CopyRight2 : Subsystem  Description=|  mask(Copyright Information){none=on}
      | Copyright info block.                                               
      |                                                                     
      | Place copyright information at the top of every subsystem in design.
      mask prompts: none "No parameters"
      mask help: Place copyright information at the top of every subsystem in design.
      mask Display:
      | NxtrConf = 'Nexteer Confidential';
      | 
      | sys = bdroot; %handle for the current model ("system")
      | first = get_param(sys,'Created');
      | first = first(end-3:end);  %year is last four digits
      | 
      | last = get_param(sys,'LastModifiedDate');
      | if isempty(last)
      |     last = datestr(now,'yyyy');
      | else
      |     last = last(end-3:end);
      | end
      | 
      | if strcmp(first,last)
      |     fprintf('%s -- Copyright %s Nexteer',NxtrConf,first)
      | else
      |     fprintf('%s -- %s%s- %s Nexteer',NxtrConf,char(169),first,last)
      | end
  Terminator : Terminator
  wires:
  PinSt/1 -> Terminator/1

== system ES004A_PwrUpSeq/PwrUpSeq/PwrUpSeqInit1/CopyRight2 ==

== system ES004A_PwrUpSeq/PwrUpSeq/PwrUpSeqPer1/CopyRight2 ==

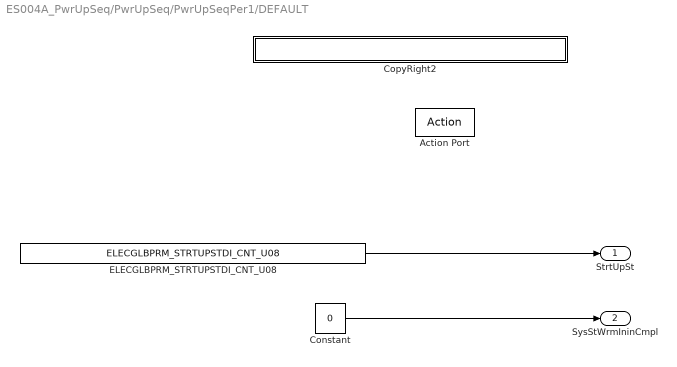
== system ES004A_PwrUpSeq/PwrUpSeq/PwrUpSeqPer1/DEFAULT ==
  Action Port : ActionPort  ActionType=default
  Constant : Constant  Value=0  OutDataTypeStr=boolean
  CopyRight2 : Subsystem  Description=|  mask(Copyright Information){none=on}
      | Copyright info block.                                               
      |                                                                     
      | Place copyright information at the top of every subsystem in design.
      mask prompts: none "No parameters"
      mask help: Place copyright information at the top of every subsystem in design.
      mask Display:
      | NxtrConf = 'Nexteer Confidential';
      | 
      | sys = bdroot; %handle for the current model ("system")
      | first = get_param(sys,'Created');
      | first = first(end-3:end);  %year is last four digits
      | 
      | last = get_param(sys,'LastModifiedDate');
      | if isempty(last)
      |     last = datestr(now,'yyyy');
      | else
      |     last = last(end-3:end);
      | end
      | 
      | if strcmp(first,last)
      |     fprintf('%s -- Copyright %s Nexteer',NxtrConf,first)
      | else
      |     fprintf('%s -- %s%s- %s Nexteer',NxtrConf,char(169),first,last)
      | end
  ELECGLBPRM_STRTUPSTDI_CNT_U08 : Constant  RequirementInfo="{'linktype_rmi_doors' '0000c463 (/ESG Group/FDD Module Requirements/EA4 Specific/ES004A_PowerUpSeq)' '#ES004A_92' 'true' 'REQ:  ES004A_92' '' } %GIDa_3597ee02_1051_49da_9cc1_a1bd3f94ea25"  Value=ELECGLBPRM_STRTUPSTDI_CNT_U08
  StrtUpSt : Outport
  SysStWrmIninCmpl : Outport  Port=2
  wires:
  Constant/1 -> SysStWrmIninCmpl/1
  ELECGLBPRM_STRTUPSTDI_CNT_U08/1 -> StrtUpSt/1

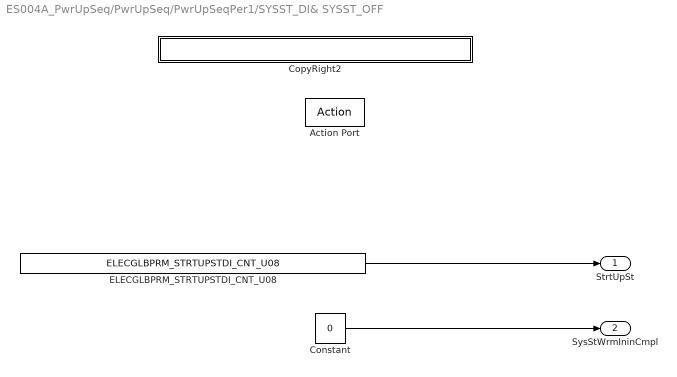
== system ES004A_PwrUpSeq/PwrUpSeq/PwrUpSeqPer1/SYSST_DI& SYSST_OFF ==
  Action Port : ActionPort  ActionType=case
  Constant : Constant  Value=0  OutDataTypeStr=boolean
  CopyRight2 : Subsystem  Description=|  mask(Copyright Information){none=on}
      | Copyright info block.                                               
      |                                                                     
      | Place copyright information at the top of every subsystem in design.
      mask prompts: none "No parameters"
      mask help: Place copyright information at the top of every subsystem in design.
      mask Display:
      | NxtrConf = 'Nexteer Confidential';
      | 
      | sys = bdroot; %handle for the current model ("system")
      | first = get_param(sys,'Created');
      | first = first(end-3:end);  %year is last four digits
      | 
      | last = get_param(sys,'LastModifiedDate');
      | if isempty(last)
      |     last = datestr(now,'yyyy');
      | else
      |     last = last(end-3:end);
      | end
      | 
      | if strcmp(first,last)
      |     fprintf('%s -- Copyright %s Nexteer',NxtrConf,first)
      | else
      |     fprintf('%s -- %s%s- %s Nexteer',NxtrConf,char(169),first,last)
      | end
  ELECGLBPRM_STRTUPSTDI_CNT_U08 : Constant  RequirementInfo="{'linktype_rmi_doors' '0000c463 (/ESG Group/FDD Module Requirements/EA4 Specific/ES004A_PowerUpSeq)' '#ES004A_92' 'true' 'REQ:  ES004A_92' '' } %GIDa_87f87ac4_a31d_47f8_aeca_77f2e092630c"  Value=ELECGLBPRM_STRTUPSTDI_CNT_U08
  StrtUpSt : Outport
  SysStWrmIninCmpl : Outport  Port=2
  wires:
  Constant/1 -> SysStWrmIninCmpl/1
  ELECGLBPRM_STRTUPSTDI_CNT_U08/1 -> StrtUpSt/1

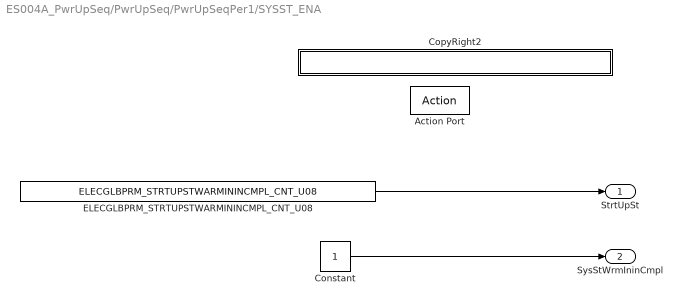
== system ES004A_PwrUpSeq/PwrUpSeq/PwrUpSeqPer1/SYSST_ENA ==
  Action Port : ActionPort  ActionType=case
  Constant : Constant  OutDataTypeStr=boolean
  CopyRight2 : Subsystem  Description=|  mask(Copyright Information){none=on}
      | Copyright info block.                                               
      |                                                                     
      | Place copyright information at the top of every subsystem in design.
      mask prompts: none "No parameters"
      mask help: Place copyright information at the top of every subsystem in design.
      mask Display:
      | NxtrConf = 'Nexteer Confidential';
      | 
      | sys = bdroot; %handle for the current model ("system")
      | first = get_param(sys,'Created');
      | first = first(end-3:end);  %year is last four digits
      | 
      | last = get_param(sys,'LastModifiedDate');
      | if isempty(last)
      |     last = datestr(now,'yyyy');
      | else
      |     last = last(end-3:end);
      | end
      | 
      | if strcmp(first,last)
      |     fprintf('%s -- Copyright %s Nexteer',NxtrConf,first)
      | else
      |     fprintf('%s -- %s%s- %s Nexteer',NxtrConf,char(169),first,last)
      | end
  ELECGLBPRM_STRTUPSTWARMININCMPL_CNT_U08 : Constant  RequirementInfo="{'linktype_rmi_doors' '0000c463 (/ESG Group/FDD Module Requirements/EA4 Specific/ES004A_PowerUpSeq)' '#ES004A_91' 'true' 'REQ:  ES004A_91' '' } %GIDa_1db9f596_d7fb_4f55_93ba_0bdf2c311370"  Value=ELECGLBPRM_STRTUPSTWARMININCMPL_CNT_U08
  StrtUpSt : Outport
  SysStWrmIninCmpl : Outport  Port=2
  wires:
  ELECGLBPRM_STRTUPSTWARMININCMPL_CNT_U08/1 -> StrtUpSt/1
  Constant/1 -> SysStWrmIninCmpl/1

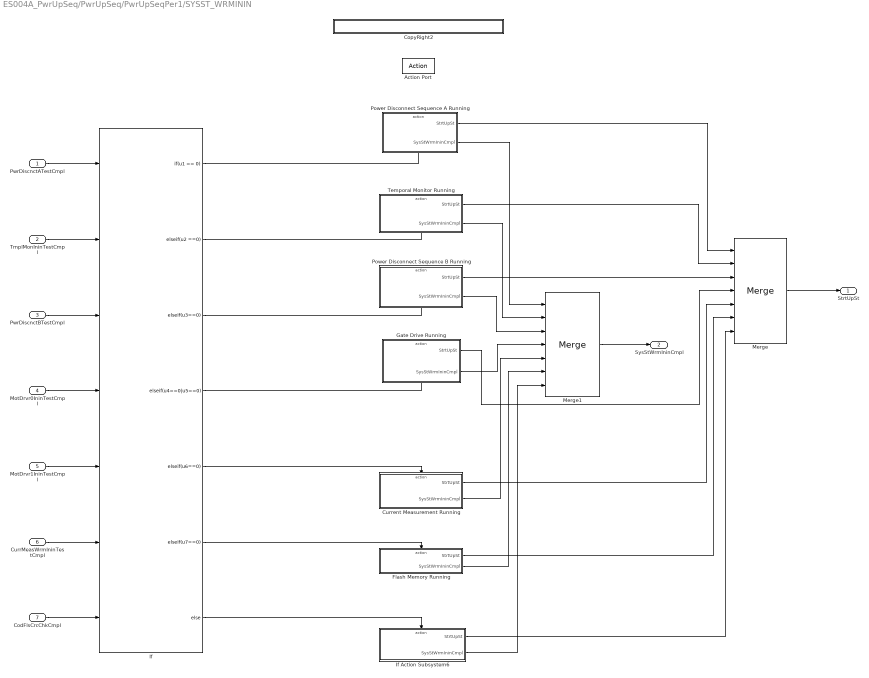
== system ES004A_PwrUpSeq/PwrUpSeq/PwrUpSeqPer1/SYSST_WRMININ ==
  PwrDiscnctATestCmpl : Inport
  TmplMonIninTestCmpl : Inport  Port=2
  PwrDiscnctBTestCmpl : Inport  Port=3
  MotDrvr0IninTestCmpl : Inport  Port=4
  MotDrvr1IninTestCmpl : Inport  Port=5
  "CurrMeasWrmIninTestCmpl " : Inport  Port=6
  CodFlsCrcChkCmpl : Inport  Port=7
  Action Port : ActionPort  ActionType=case
  CopyRight2 : Subsystem  Description=|  mask(Copyright Information){none=on}
      | Copyright info block.                                               
      |                                                                     
      | Place copyright information at the top of every subsystem in design.
      mask prompts: none "No parameters"
      mask help: Place copyright information at the top of every subsystem in design.
      mask Display:
      | NxtrConf = 'Nexteer Confidential';
      | 
      | sys = bdroot; %handle for the current model ("system")
      | first = get_param(sys,'Created');
      | first = first(end-3:end);  %year is last four digits
      | 
      | last = get_param(sys,'LastModifiedDate');
      | if isempty(last)
      |     last = datestr(now,'yyyy');
      | else
      |     last = last(end-3:end);
      | end
      | 
      | if strcmp(first,last)
      |     fprintf('%s -- Copyright %s Nexteer',NxtrConf,first)
      | else
      |     fprintf('%s -- %s%s- %s Nexteer',NxtrConf,char(169),first,last)
      | end
  Current Measurement Running : Subsystem  RequirementInfo="{'linktype_rmi_doors' '0000c463 (/ESG Group/FDD Module Requirements/EA4 Specific/ES004A_PowerUpSeq)' '#ES004A_81' 'true' 'REQ:  ES004A_81' '' } %GIDa_9127bcc1_cc29_496f_abb9_5387f3218dce"  TreatAsAtomicUnit=on
  Flash Memory Running : Subsystem  RequirementInfo="{'linktype_rmi_doors' '0000c463 (/ESG Group/FDD Module Requirements/EA4 Specific/ES004A_PowerUpSeq)' '#ES004A_83' 'true' 'REQ:  ES004A_83' '' } %GIDa_223a8b58_1f32_4b75_8519_612209f8a0b7"  TreatAsAtomicUnit=on
  Gate Drive Running : Subsystem  RequirementInfo="{'linktype_rmi_doors' '0000c463 (/ESG Group/FDD Module Requirements/EA4 Specific/ES004A_PowerUpSeq)' '#ES004A_79' 'true' 'REQ:  ES004A_79' '' } %GIDa_fa97780b_ce37_4938_a56c_a249d8282fc4"  TreatAsAtomicUnit=on
  If : If  RequirementInfo="{'linktype_rmi_doors' '0000c463 (/ESG Group/FDD Module Requirements/EA4 Specific/ES004A_PowerUpSeq)' '#ES004A_77' 'true' 'REQ:  ES004A_77' '' ; 'linktype_rmi_doors' '0000c463 (/ESG Group/FDD Module Requirements/EA4 Specific/ES004A_PowerUpSeq)' '#ES004A_78' 'true' 'REQ:  ES004A_78' '' ; 'linktype_rmi_doors' '0000c463 (/ESG Group/FDD Module Requirements/EA4 Specific/ES004A_PowerUpSeq)' '#ES004A_78' 'true' 'REQ:  ES004A_78' '' ; 'linktype_rmi_doors' '0000c463 (/ESG Group/FDD Module Requirements/EA4 Specific/ES004A_PowerUpSeq)' '#ES004A_79' 'true' 'REQ:  ES004A_79' '' ; 'linktype_rmi_doors' '0000c463 (/ESG Group/FDD Module Requirements/EA4 Specific/ES004A_PowerUpSeq)' '#ES004A_81' 'true' 'REQ:  ES004A_81' '' ; 'linktype_rmi_doors' '0000c463 (/ESG Group/FDD Module Requirements/EA4 Specific/ES004A_PowerUpSeq)' '#ES004A_83' 'true' 'REQ:  ES004A_83' '' ; 'linktype_rmi_doors' '0000c463 (/ESG Group/FDD Module Requirements/EA4 Specific/ES004A_PowerUpSeq)' '#ES004A_110' 'true' 'REQ:  ES004A_110' '' } %GIDa_cc1f6fd8_f4d8_407b_adba_65b9339b7100"  NumInputs=7  IfExpression=u1 == 0  ElseIfExpressions=u2 ==0 , u3==0 ,u4==0|u5==0,u6==0 ,u7==0
  If Action Subsystem6 : Subsystem  RequirementInfo="{'linktype_rmi_doors' '0000c463 (/ESG Group/FDD Module Requirements/EA4 Specific/ES004A_PowerUpSeq)' '#ES004A_110' 'true' 'REQ:  ES004A_110' '' } %GIDa_80ed37f1_ece5_4513_b447_e96ba05333ff"  TreatAsAtomicUnit=on
  Merge : Merge  RequirementInfo={} %GIDa_122839eb_5789_49ce_b5d2_bbf350e44528  Inputs=7
  Merge1 : Merge  RequirementInfo={} %GIDa_6a46f8bd_5f76_4d3c_9220_efb51c651a60  Inputs=7
  Power Disconnect Sequence A Running : Subsystem  RequirementInfo="{'linktype_rmi_doors' '0000c463 (/ESG Group/FDD Module Requirements/EA4 Specific/ES004A_PowerUpSeq)' '#ES004A_82' 'true' 'REQ:  ES004A_82' '' } %GIDa_c8935141_a908_4031_b016_5fc8ea4342bc"  TreatAsAtomicUnit=on
  Power Disconnect Sequence B Running : Subsystem  RequirementInfo="{'linktype_rmi_doors' '0000c463 (/ESG Group/FDD Module Requirements/EA4 Specific/ES004A_PowerUpSeq)' '#ES004A_78' 'true' 'REQ:  ES004A_78' '' } %GIDa_0ffc4163_1829_483d_be03_50a27c61aff4"  TreatAsAtomicUnit=on
  Temporal Monitor Running : Subsystem  RequirementInfo="{'linktype_rmi_doors' '0000c463 (/ESG Group/FDD Module Requirements/EA4 Specific/ES004A_PowerUpSeq)' '#ES004A_77' 'true' 'REQ:  ES004A_77' '' } %GIDa_acc93fdb_524a_4561_ac59_7d6169685fa0"  TreatAsAtomicUnit=on
  StrtUpSt : Outport  RequirementInfo="{'linktype_rmi_doors' '0000c463 (/ESG Group/FDD Module Requirements/EA4 Specific/ES004A_PowerUpSeq)' '#ES004A_55' 'true' 'REQ:  ES004A_55' '' } %GIDa_8fb86dbe_1acd_4e28_b2c1_efdddb0b395e"
  SysStWrmIninCmpl : Outport  Port=2
  wires:
  PwrDiscnctATestCmpl/1 -> If/1
  TmplMonIninTestCmpl/1 -> If/2
  PwrDiscnctBTestCmpl/1 -> If/3
  MotDrvr0IninTestCmpl/1 -> If/4
  "CurrMeasWrmIninTestCmpl "/1 -> If/6
  CodFlsCrcChkCmpl/1 -> If/7
  If/1 -> Power Disconnect Sequence A Running/Action
  If/2 -> Temporal Monitor Running/Action
  If/3 -> Power Disconnect Sequence B Running/Action
  If/4 -> Gate Drive Running/Action
  If/5 -> Current Measurement Running/Action
  If/6 -> Flash Memory Running/Action
  If/7 -> If Action Subsystem6/Action
  Merge1/1 -> SysStWrmIninCmpl/1
  Merge/1 -> StrtUpSt/1
  MotDrvr1IninTestCmpl/1 -> If/5
  Power Disconnect Sequence A Running/2(SysStWrmIninCmpl) -> Merge1/1
  Temporal Monitor Running/2(SysStWrmIninCmpl) -> Merge1/2
  Power Disconnect Sequence B Running/2(SysStWrmIninCmpl) -> Merge1/3
  Gate Drive Running/2(SysStWrmIninCmpl) -> Merge1/4
  Current Measurement Running/2(SysStWrmIninCmpl) -> Merge1/5
  Flash Memory Running/2(SysStWrmIninCmpl) -> Merge1/6
  If Action Subsystem6/2(SysStWrmIninCmpl) -> Merge1/7
  Power Disconnect Sequence A Running/1(StrtUpSt) -> Merge/1
  Temporal Monitor Running/1(StrtUpSt) -> Merge/2
  Power Disconnect Sequence B Running/1(StrtUpSt) -> Merge/3
  Gate Drive Running/1(StrtUpSt) -> Merge/4
  Current Measurement Running/1(StrtUpSt) -> Merge/5
  Flash Memory Running/1(StrtUpSt) -> Merge/6
  If Action Subsystem6/1(StrtUpSt) -> Merge/7

== system ES004A_PwrUpSeq/PwrUpSeq/PwrUpSeqPer1/SetTODHighState  ==
  note: Note:
      | PwrTurnOffCtrl is a SrvRunnable for thios component
      | so can be called as a local function in the software.
  Enable : EnablePort
  Constant : Constant  OutDataTypeStr=boolean
  CopyRight2 : Subsystem  Description=|  mask(Copyright Information){none=on}
      | Copyright info block.                                               
      |                                                                     
      | Place copyright information at the top of every subsystem in design.
      mask prompts: none "No parameters"
      mask help: Place copyright information at the top of every subsystem in design.
      mask Display:
      | NxtrConf = 'Nexteer Confidential';
      | 
      | sys = bdroot; %handle for the current model ("system")
      | first = get_param(sys,'Created');
      | first = first(end-3:end);  %year is last four digits
      | 
      | last = get_param(sys,'LastModifiedDate');
      | if isempty(last)
      |     last = datestr(now,'yyyy');
      | else
      |     last = last(end-3:end);
      | end
      | 
      | if strcmp(first,last)
      |     fprintf('%s -- Copyright %s Nexteer',NxtrConf,first)
      | else
      |     fprintf('%s -- %s%s- %s Nexteer',NxtrConf,char(169),first,last)
      | end
  PwrTurnOffCtrl : Subsystem  TreatAsAtomicUnit=on
  wires:
  Constant/1 -> PwrTurnOffCtrl/1(PwrTurnOffCtrl_ArgIn)

== system ES004A_PwrUpSeq/PwrUpSeq/PwrTurnOffCtrl/IoHwAb_SetGpioPwrTurnOffCtrl/CopyRight2 ==

== system ES004A_PwrUpSeq/PwrUpSeq/PwrUpSeqPer1/DEFAULT/CopyRight2 ==

== system ES004A_PwrUpSeq/PwrUpSeq/PwrUpSeqPer1/SYSST_DI& SYSST_OFF/CopyRight2 ==

== system ES004A_PwrUpSeq/PwrUpSeq/PwrUpSeqPer1/SYSST_ENA/CopyRight2 ==

== system ES004A_PwrUpSeq/PwrUpSeq/PwrUpSeqPer1/SYSST_WRMININ/CopyRight2 ==

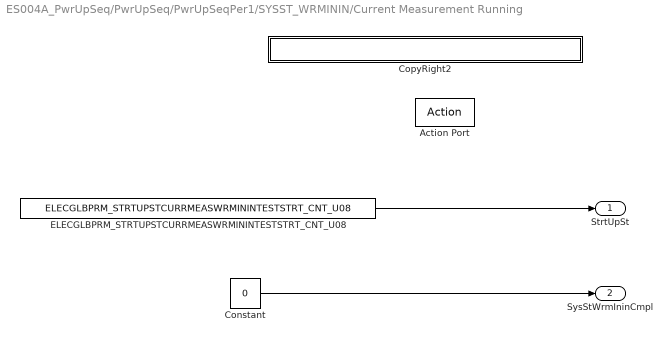
== system ES004A_PwrUpSeq/PwrUpSeq/PwrUpSeqPer1/SYSST_WRMININ/Current Measurement Running ==
  Action Port : ActionPort  ActionType=elseif
  Constant : Constant  Value=0  OutDataTypeStr=boolean
  CopyRight2 : Subsystem  Description=|  mask(Copyright Information){none=on}
      | Copyright info block.                                               
      |                                                                     
      | Place copyright information at the top of every subsystem in design.
      mask prompts: none "No parameters"
      mask help: Place copyright information at the top of every subsystem in design.
      mask Display:
      | NxtrConf = 'Nexteer Confidential';
      | 
      | sys = bdroot; %handle for the current model ("system")
      | first = get_param(sys,'Created');
      | first = first(end-3:end);  %year is last four digits
      | 
      | last = get_param(sys,'LastModifiedDate');
      | if isempty(last)
      |     last = datestr(now,'yyyy');
      | else
      |     last = last(end-3:end);
      | end
      | 
      | if strcmp(first,last)
      |     fprintf('%s -- Copyright %s Nexteer',NxtrConf,first)
      | else
      |     fprintf('%s -- %s%s- %s Nexteer',NxtrConf,char(169),first,last)
      | end
  ELECGLBPRM_STRTUPSTCURRMEASWRMININTESTSTRT_CNT_U08 : Constant  RequirementInfo="{'linktype_rmi_doors' '0000c463 (/ESG Group/FDD Module Requirements/EA4 Specific/ES004A_PowerUpSeq)' '#ES004A_90' 'true' 'REQ:  ES004A_90' '' } %GIDa_0e2887c5_0a04_45c7_936a_f5bd77c94aac"  Value=ELECGLBPRM_STRTUPSTCURRMEASWRMININTESTSTRT_CNT_U08
  StrtUpSt : Outport
  SysStWrmIninCmpl : Outport  Port=2
  wires:
  ELECGLBPRM_STRTUPSTCURRMEASWRMININTESTSTRT_CNT_U08/1 -> StrtUpSt/1
  Constant/1 -> SysStWrmIninCmpl/1

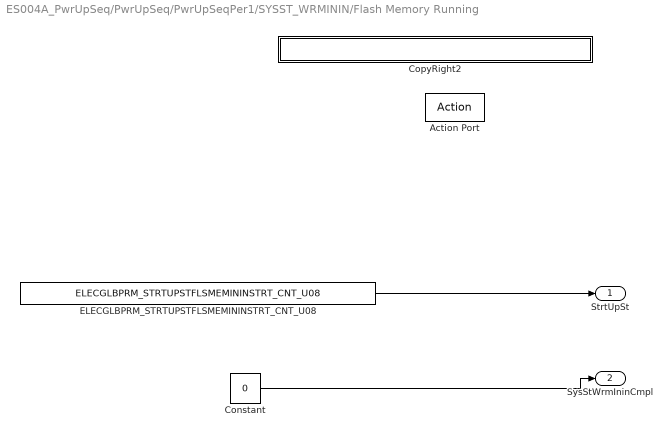
== system ES004A_PwrUpSeq/PwrUpSeq/PwrUpSeqPer1/SYSST_WRMININ/Flash Memory Running ==
  Action Port : ActionPort  ActionType=elseif
  Constant : Constant  Value=0  OutDataTypeStr=boolean
  CopyRight2 : Subsystem  Description=|  mask(Copyright Information){none=on}
      | Copyright info block.                                               
      |                                                                     
      | Place copyright information at the top of every subsystem in design.
      mask prompts: none "No parameters"
      mask help: Place copyright information at the top of every subsystem in design.
      mask Display:
      | NxtrConf = 'Nexteer Confidential';
      | 
      | sys = bdroot; %handle for the current model ("system")
      | first = get_param(sys,'Created');
      | first = first(end-3:end);  %year is last four digits
      | 
      | last = get_param(sys,'LastModifiedDate');
      | if isempty(last)
      |     last = datestr(now,'yyyy');
      | else
      |     last = last(end-3:end);
      | end
      | 
      | if strcmp(first,last)
      |     fprintf('%s -- Copyright %s Nexteer',NxtrConf,first)
      | else
      |     fprintf('%s -- %s%s- %s Nexteer',NxtrConf,char(169),first,last)
      | end
  ELECGLBPRM_STRTUPSTFLSMEMININSTRT_CNT_U08 : Constant  RequirementInfo="{'linktype_rmi_doors' '0000c463 (/ESG Group/FDD Module Requirements/EA4 Specific/ES004A_PowerUpSeq)' '#ES004A_105' 'true' 'REQ:  ES004A_105' '' } %GIDa_6d003dc2_d186_41c9_ae1c_92ef3d36c34c"  Value=ELECGLBPRM_STRTUPSTFLSMEMININSTRT_CNT_U08
  StrtUpSt : Outport
  SysStWrmIninCmpl : Outport  Port=2
  wires:
  ELECGLBPRM_STRTUPSTFLSMEMININSTRT_CNT_U08/1 -> StrtUpSt/1
  Constant/1 -> SysStWrmIninCmpl/1

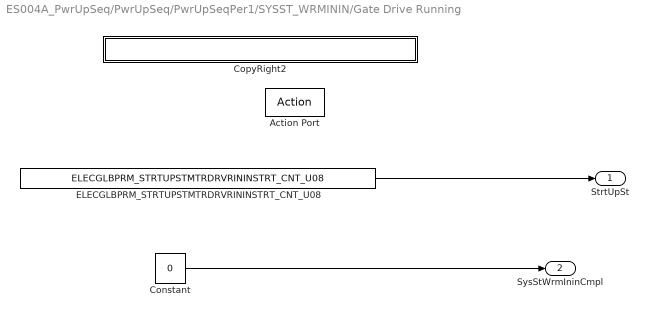
== system ES004A_PwrUpSeq/PwrUpSeq/PwrUpSeqPer1/SYSST_WRMININ/Gate Drive Running ==
  Action Port : ActionPort  ActionType=elseif
  Constant : Constant  Value=0  OutDataTypeStr=boolean
  CopyRight2 : Subsystem  Description=|  mask(Copyright Information){none=on}
      | Copyright info block.                                               
      |                                                                     
      | Place copyright information at the top of every subsystem in design.
      mask prompts: none "No parameters"
      mask help: Place copyright information at the top of every subsystem in design.
      mask Display:
      | NxtrConf = 'Nexteer Confidential';
      | 
      | sys = bdroot; %handle for the current model ("system")
      | first = get_param(sys,'Created');
      | first = first(end-3:end);  %year is last four digits
      | 
      | last = get_param(sys,'LastModifiedDate');
      | if isempty(last)
      |     last = datestr(now,'yyyy');
      | else
      |     last = last(end-3:end);
      | end
      | 
      | if strcmp(first,last)
      |     fprintf('%s -- Copyright %s Nexteer',NxtrConf,first)
      | else
      |     fprintf('%s -- %s%s- %s Nexteer',NxtrConf,char(169),first,last)
      | end
  ELECGLBPRM_STRTUPSTMTRDRVRININSTRT_CNT_U08 : Constant  RequirementInfo="{'linktype_rmi_doors' '0000c463 (/ESG Group/FDD Module Requirements/EA4 Specific/ES004A_PowerUpSeq)' '#ES004A_89' 'true' 'REQ:  ES004A_89' '' } %GIDa_36727618_0b71_4f5b_9cad_ec55d2d38298"  Value=ELECGLBPRM_STRTUPSTMTRDRVRININSTRT_CNT_U08
  StrtUpSt : Outport
  SysStWrmIninCmpl : Outport  Port=2
  wires:
  ELECGLBPRM_STRTUPSTMTRDRVRININSTRT_CNT_U08/1 -> StrtUpSt/1
  Constant/1 -> SysStWrmIninCmpl/1

== system ES004A_PwrUpSeq/PwrUpSeq/PwrUpSeqPer1/SYSST_WRMININ/If Action Subsystem6 ==
  Action Port : ActionPort  ActionType=else
  Constant : Constant  RequirementInfo="{'linktype_rmi_doors' '0000c463 (/ESG Group/FDD Module Requirements/EA4 Specific/ES004A_PowerUpSeq)' '#ES004A_62' 'true' 'REQ:  ES004A_62' '' } %GIDa_ef0c3e1b_e774_45f1_88e7_90c323b093a0"  OutDataTypeStr=boolean
  CopyRight2 : Subsystem  Description=|  mask(Copyright Information){none=on}
      | Copyright info block.                                               
      |                                                                     
      | Place copyright information at the top of every subsystem in design.
      mask prompts: none "No parameters"
      mask help: Place copyright information at the top of every subsystem in design.
      mask Display:
      | NxtrConf = 'Nexteer Confidential';
      | 
      | sys = bdroot; %handle for the current model ("system")
      | first = get_param(sys,'Created');
      | first = first(end-3:end);  %year is last four digits
      | 
      | last = get_param(sys,'LastModifiedDate');
      | if isempty(last)
      |     last = datestr(now,'yyyy');
      | else
      |     last = last(end-3:end);
      | end
      | 
      | if strcmp(first,last)
      |     fprintf('%s -- Copyright %s Nexteer',NxtrConf,first)
      | else
      |     fprintf('%s -- %s%s- %s Nexteer',NxtrConf,char(169),first,last)
      | end
  ELECGLBPRM_STRTUPSTWARMININCMPL_CNT_U08 : Constant  RequirementInfo="{'linktype_rmi_doors' '0000c463 (/ESG Group/FDD Module Requirements/EA4 Specific/ES004A_PowerUpSeq)' '#ES004A_91' 'true' 'REQ:  ES004A_91' '' } %GIDa_e5d51196_a843_4f31_946c_3457520e7be2"  Value=ELECGLBPRM_STRTUPSTWARMININCMPL_CNT_U08
  StrtUpSt : Outport
  SysStWrmIninCmpl : Outport  Port=2
  wires:
  ELECGLBPRM_STRTUPSTWARMININCMPL_CNT_U08/1 -> StrtUpSt/1
  Constant/1 -> SysStWrmIninCmpl/1

== system ES004A_PwrUpSeq/PwrUpSeq/PwrUpSeqPer1/SYSST_WRMININ/Power Disconnect Sequence A Running ==
  Action Port : ActionPort  ActionType=then
  Constant : Constant  RequirementInfo="{'linktype_rmi_doors' '0000c463 (/ESG Group/FDD Module Requirements/EA4 Specific/ES004A_PowerUpSeq)' '#ES004A_63' 'true' 'REQ:  ES004A_63' '' } %GIDa_1ac0845e_d558_4790_a0f1_f566be7b5692"  Value=0  OutDataTypeStr=boolean
  CopyRight2 : Subsystem  Description=|  mask(Copyright Information){none=on}
      | Copyright info block.                                               
      |                                                                     
      | Place copyright information at the top of every subsystem in design.
      mask prompts: none "No parameters"
      mask help: Place copyright information at the top of every subsystem in design.
      mask Display:
      | NxtrConf = 'Nexteer Confidential';
      | 
      | sys = bdroot; %handle for the current model ("system")
      | first = get_param(sys,'Created');
      | first = first(end-3:end);  %year is last four digits
      | 
      | last = get_param(sys,'LastModifiedDate');
      | if isempty(last)
      |     last = datestr(now,'yyyy');
      | else
      |     last = last(end-3:end);
      | end
      | 
      | if strcmp(first,last)
      |     fprintf('%s -- Copyright %s Nexteer',NxtrConf,first)
      | else
      |     fprintf('%s -- %s%s- %s Nexteer',NxtrConf,char(169),first,last)
      | end
  ELECGLBPRM_STRTUPSTPWRDISCNCTATESTSTRT_CNT_U08 : Constant  RequirementInfo="{'linktype_rmi_doors' '0000c463 (/ESG Group/FDD Module Requirements/EA4 Specific/ES004A_PowerUpSeq)' '#ES004A_86' 'true' 'REQ:  ES004A_86' '' } %GIDa_dae88499_1855_4a7d_a695_1a0cb350f1f9"  Value=ELECGLBPRM_STRTUPSTPWRDISCNCTATESTSTRT_CNT_U08
  StrtUpSt : Outport
  SysStWrmIninCmpl : Outport  Port=2
  wires:
  ELECGLBPRM_STRTUPSTPWRDISCNCTATESTSTRT_CNT_U08/1 -> StrtUpSt/1
  Constant/1 -> SysStWrmIninCmpl/1
